simulink model "readArray2"  (R2012b)
settings: Solver=FixedStepDiscrete  SolverMode=MultiTasking  StartTime=0.0  StopTime=10.0  FixedStep=0.001  RelTol=1e-3
undefined symbols (not defined in the file): macaddr, modelConstants, mxpcnbunlink, rereferencingType
libraries: xpcnetworkbufferlib x2, xpcethernetlib x2, simulink x1
settings Model: xpc_rtwmakecfg_data=_xpcetherlib__xpcether8255xlib__xpcetherGbElib__xpcnblib_  BufferReuse=off  Creator=gilja  LastModifiedBy=NPTL
settings SolverCC: EnableConcurrentExecution=on  ConcurrentTasks=on
settings DataIOCC: SaveOutput=off  SignalLogging=off  DSMLogging=off  SaveTime=off
settings OptimizationCC: BlockReduction=off  InlineParams=on  InlineInvariantSignals=on  OptimizeBlockIOStorage=off  BufferReuse=off  ExpressionFolding=off  LocalBlockOutputs=off
settings HardwareCC: ProdIntDivRoundTo=Zero  ProdEndianess=LittleEndian  ProdHWDeviceType=Generic->32-bit x86 compatible
settings ModelReferenceCC: ModelReferenceNumInstancesAllowed=Single  PropagateVarSize=During execution  ModelReferenceMinAlgLoopOccurrences=on
settings SFSimCC: SimCustomHeaderCode="#include \"cerebusParse.h\""  SimUserSources=cerebusParse.c  SimUserIncludeDirs=C:\Progra~1\MATLAB\R2012b\toolbox\rtw\targets\xpc\target\build\xpcblocks\include
settings RTWCC: SystemTargetFile=xpctarget.tlc  TemplateMakefile=xpc_default_tmf  Description=xPC Target  ProcessScript=xpctarget_make_rtw_hook  RTWUseSimCustomCode=on  CustomHeaderCode="#include \"cerebusParse.h\""  CustomInclude=C:\Progra~1\MATLAB\R2012b\toolbox\rtw\targets\xpc\target\build\xpcblocks\include  CustomSource=cerebusParse.c  RTWCompilerOptimization=On
settings CodeAppCC: MaxIdLength=62
settings xpcTargetCC: TargetFcnLib=ansi_tfl_table_tmw.mat  CodeReplacementLibrary=XPC_BLAS  ParMdlRefBuildCompliant=on  ConcurrentExecutionCompliant=on  CombineSignalStateStructs=off  GRTInterface=on  xPCTaskExecutionProfile=on  xPCRL32EventNumber=5000  xPCisDownloadable=off  xPCLoadParamSetFile=off  xPCConcurrentTasks=off  xPCEnableSFAnimation=off

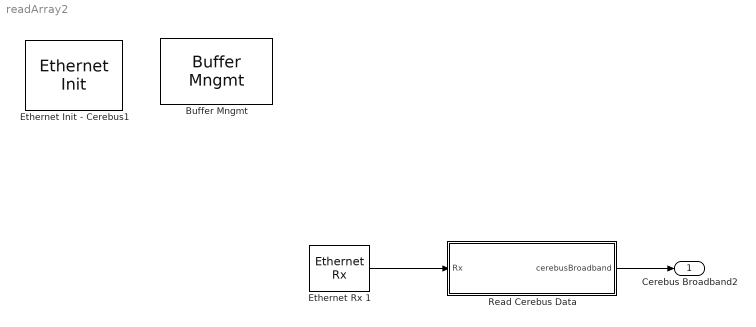
== system readArray2 ==
  "Buffer Mngmt " : xpcnetworkbufferlib/Buffer Mngmt   Priority=-1  SampleTime=-1  PoolSizes=modelConstants.networkBufferPoolSizes  ShowTune=on
  Ethernet Init - Cerebus1 : xpcethernetlib/Ethernet Init   Priority=-1  ID=5  Driver=Intel Gigabit  Bus=modelConstants.xpcNICConfig.nsp2.bus  Slot=modelConstants.xpcNICConfig.nsp2.slot  SampleTime=-1  AddressSource=Specify  MAC=macaddr('00:00:00:00:00:00')  TxSA=off  RxPromiscuous=off  Multicast={}  RxBad=off  RxShort=off  MaxMTU=1518  TxThreshold=10  TxBuffers=128  RxBuffers=64  ShowTune=on  NumRxBlks=1
  Ethernet Rx 1 : xpcethernetlib/Ethernet Rx   ID=5  SampleTime=modelConstants.sampleTime  Criteria=Receive all unmatched types [0 to 65535]  EtherType=[hex2dec('0000')]  BlkID=0
  Read Cerebus Data : Subsystem
  Cerebus Broadband2 : Outport  OutDataTypeStr=Bus: cerebusBroadband  BusOutputAsStruct=on
  wires:
  Ethernet Rx 1/1 -> Read Cerebus Data/1(Rx)
  Read Cerebus Data/1(cerebusBroadband) -> Cerebus Broadband2/1

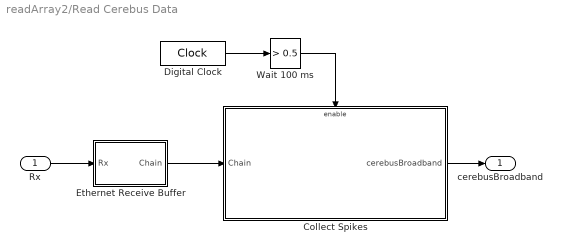
== system readArray2/Read Cerebus Data ==
  Rx : Inport
  Collect Spikes : Subsystem
  Digital Clock : DigitalClock  SampleTime=0.001
  Ethernet Receive Buffer : Subsystem
  Wait 100 ms : simulink/Logic and Bit Operations/Compare To Constant  relop=>  const=0.5  OutDataTypeStr=boolean
  cerebusBroadband : Outport  OutDataTypeStr=Bus: cerebusBroadband
  wires:
  Collect Spikes/1(cerebusBroadband) -> cerebusBroadband/1
  Wait 100 ms/1 -> Collect Spikes/Enable
  Digital Clock/1 -> Wait 100 ms/1
  Ethernet Receive Buffer/1(Chain) -> Collect Spikes/1(Chain)
  Rx/1 -> Ethernet Receive Buffer/1(Rx)

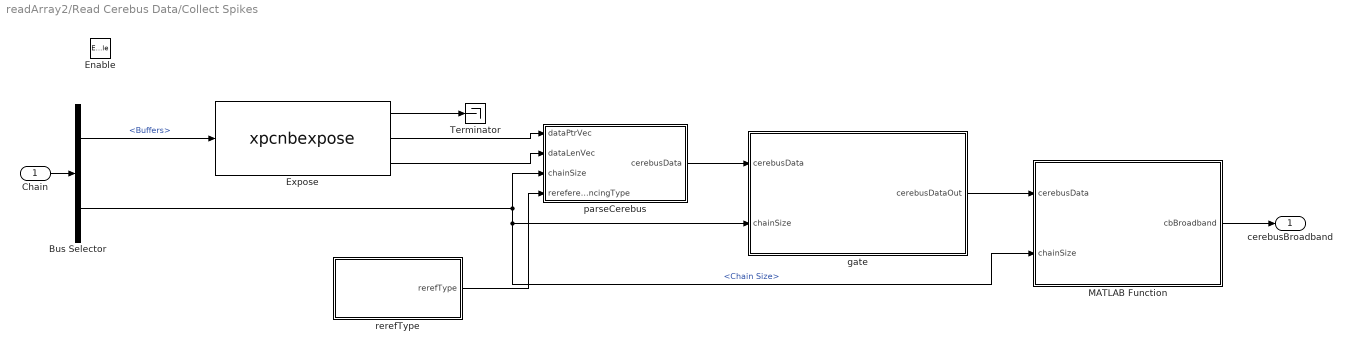
== system readArray2/Read Cerebus Data/Collect Spikes ==
  Chain : Inport
  Enable : EnablePort  StatesWhenEnabling=reset  PropagateVarSize=During execution
  Bus Selector : BusSelector  OutputSignals=Buffers,Chain Size
  Expose : S-Function  InitFcn=mxpcnbunlink(1,0);  FunctionName=xpcnbexpose  Parameters=vectorLength  EnableBusSupport=off  mask(xpcnbunlink){VectorLength=50}
      mask prompts: VectorLength "Vector length (-1 inherit):"
      mask help: Network Buffer Exposure
      mask init:
      | [vectorLength] = mxpcnbunlink(2, VectorLength);
      mask Help: eval('xpcdoc(''NB_Unlink'')');
      mask Display:
      | disp('NB Expose');
      | port_label('output', 1, 'NBVec');
      | port_label('output', 2, 'DataPtrVec');
      | port_label('output', 3, 'DataLenVec');
  MATLAB Function : MATLAB Function  TreatAsAtomicUnit=on
  Terminator : Terminator
  gate : MATLAB Function  TreatAsAtomicUnit=on
  parseCerebus : MATLAB Function  TreatAsAtomicUnit=on
  rerefType : Subsystem
  cerebusBroadband : Outport  OutDataTypeStr=Bus: cerebusBroadband
  wires:
  gate/1(cerebusDataOut) -> MATLAB Function/1(cerebusData)
  Chain/1 -> Bus Selector/1
  MATLAB Function/1(cbBroadband) -> cerebusBroadband/1
  Bus Selector/1 -> Expose/1  "<Buffers>"
  Expose/2 -> parseCerebus/1(dataPtrVec)
  Expose/3 -> parseCerebus/2(dataLenVec)
  Bus Selector/2 -> parseCerebus/3(chainSize), MATLAB Function/2(chainSize), gate/2(chainSize)  "<Chain Size>"
  parseCerebus/1(cerebusData) -> gate/1(cerebusData)
  Expose/1 -> Terminator/1
  rerefType/1(rerefType) -> parseCerebus/4(rereferencingType)

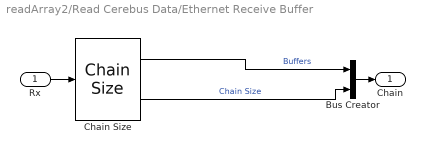
== system readArray2/Read Cerebus Data/Ethernet Receive Buffer ==
  Rx : Inport
  Bus Creator : BusCreator  Inputs=2
  "Chain Size " : xpcnetworkbufferlib/Chain Size 
  Chain : Outport
  wires:
  Rx/1 -> "Chain Size "/1
  "Chain Size "/2 -> Bus Creator/2  "Chain Size"
  Bus Creator/1 -> Chain/1
  "Chain Size "/1 -> Bus Creator/1  "Buffers"

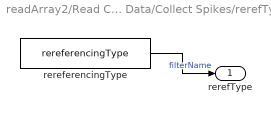
== system readArray2/Read Cerebus Data/Collect Spikes/rerefType ==
  rereferencingType : Constant  Value=rereferencingType
  rerefType : Outport
  wires:
  rereferencingType/1 -> rerefType/1  "filterName"

== matlab function readArray2/Read Cerebus Data/Collect Spikes/parseCerebus ==
  data: dataPtrVec input size=[1 50]; cerebusData output Bus: cerebusData; dataLenVec input size=[1 50]; chainSize input size=[1 1]; rereferencingType input
function cerebusData  = parseCerebus(dataPtrVec, dataLenVec, chainSize, rereferencingType)
%#codegen

    persistent lastPacketTime;
    persistent firstPacket;
    persistent contiguousInvalidGroupPackets;
    if isempty(lastPacketTime)
        lastPacketTime = uint32(0);
        firstPacket = true;
        contiguousInvalidGroupPackets = uint16(0);
    end

    %numCerebusChannels = xpcConstants.cerebus.numCerebusChannels;
    %maxSamplesInMS = xpcConstants.cerebus.maxSamplesInMS;
    %continuousGroupId = xpcConstants.cerebus.continuousGroupId;
    
    numCerebusChannels = 96;
    maxSamplesInMS = 150;
    continuousGroupId = 5;
    
    % initialize
    numSamples = uint32(0); % ideally, either 0, 30, or 60
    samples = zeros([numCerebusChannels maxSamplesInMS], 'int16');
    cerebusTimes = zeros(maxSamplesInMS, 1, 'uint32');
    
    curTime = coder.nullcopy(uint32(0));
    
    %% 
    % loop through all UDP packets that came in
    for iP = uint8(1) : uint8(chainSize)
        
        if dataPtrVec(iP) == 0 || dataLenVec(iP) == 0
            continue;
        end

        % define buffers
        pp = coder.opaque('cbPKT_GENERIC*', 'NULL');
        pBufferEnd = coder.opaque('UINT8_T*', 'NULL');
        
        % grab pointer to end of UDP packet
        pp = coder.ceval('(cbPKT_GENERIC*)', dataPtrVec(iP) + uint32(42)); % do a cast operation - +42 is for jumping over the ethernet + IP + UDP header
        pBufferEnd = coder.ceval('cb_getPointerToBufferEnd', pp, uint32(dataLenVec(iP)));
        
        %%
        % loop over all cbPkts in this UDP packet
        while true  


            isGroupPkt = coder.nullcopy(uint8(0));
            isGroupPkt = coder.ceval('cb_isContinuousPacketForGroup', pp, uint8(continuousGroupId));
                       
            if isGroupPkt
                
                % get time
                curTime = coder.nullcopy(uint32(0));
                curTime = coder.ceval('cb_getTime', pp); % uint32 cerebus timestamp

                % CP & PN - 16/09/20 avoiding bad group packets that seem to pass
                % groupId screen, yet have very odd sample times
                if firstPacket
                    firstPacket = false;
                    lastPacketTime = curTime; % last valid uint32 timestamp
                else
                    % if the packet has a weird timestamp, do not increment
                    % numsamples, do not copy into continuous samples
                    if abs( single(curTime) - single(lastPacketTime) ) < 61 % we can drop 2 ms of packets, and this screen still works
                        
                        % receieved continuous data sample for the appropriate group id
                        numSamples = numSamples + uint32(1);
                        contiguousInvalidGroupPackets = uint16(0);
                        lastPacketTime = curTime;

                        cerebusTimes(numSamples) = curTime;

                        % copy in the samples
                        coder.ceval('cb_copyContinuousSamples', pp, coder.ref(samples(1, numSamples)), size(samples, 1)); 
                        
                    else
                        
                        % got invalid group packet
                        contiguousInvalidGroupPackets = contiguousInvalidGroupPackets + uint16(1);
                        
                    end
                end
                
            end
            
            % test to ensure we didn't get a bad timestamp on the very
            % first time, otherwise will never get neural data
            if contiguousInvalidGroupPackets > uint16(100)
                contiguousInvalidGroupPackets = uint16(0);
                lastPacketTime = curTime;
            end

            % jump to the next cbPKT
            pNext = coder.nullcopy(uint8(0));
            pNext = coder.ceval('cb_hasNext', pp, pBufferEnd);
            
            if ~pNext % check to see if no more cbPkts in this UDP packet
                break; % break while
            end
            
            % update pointer to next cbPkt
            pNext = coder.opaque('cbPKT_GENERIC*', 'NULL');
            pNext = coder.ceval('cb_getNext', pp);
            pp = pNext;
            
        end  % end while loop over all cbPkts in this UDP packet
        
    end % end for loop over all UDP packets

    % apply rereferencing
    switch rereferencingType
        case rigHardwareConstants.REREFERENCE_NONE
            % no common referencing, take the values as is, do nothing here
        case rigHardwareConstants.REREFERENCE_COMMON_AVG
            % Common avg reference:
            samples(:,1:numSamples) = samples(:,1:numSamples) - int16( repmat(   mean(single(samples(:, 1:numSamples)), 1), size(samples, 1), 1) );
        case rigHardwareConstants.REREFERENCE_COMMON_MEDIAN
            % Common median reference:
            samples(:,1:numSamples) = samples(:,1:numSamples) - int16( repmat( median(single(samples(:, 1:numSamples)), 1), size(samples, 1), 1) );
    end
    
    cerebusData.numSamples = numSamples;
    cerebusData.samples = samples'; % this is time x channels
    cerebusData.sampleTimes = cerebusTimes;
    cerebusData.firstCerebusTime = cerebusTimes(1);
    cerebusData.lastCerebusTime = cerebusTimes(numSamples);

end

== matlab function readArray2/Read Cerebus Data/Collect Spikes/MATLAB Function ==
  data: cerebusData input Bus: cerebusData; cbBroadband output Bus: cerebusBroadband size=1; xpcConstants parameter; chainSize input size=[1 1]
function cbBroadband  = bufferCerebusSamples(cerebusData, xpcConstants, chainSize)
%#codegen

persistent sampleBuffer bufferInIdx bufferOutIdx outputValidP bufferInit;

numCerebusChannels = xpcConstants.cerebus.numCerebusChannels;
bufferSize = xpcConstants.cerebus.sampleBufferSize;
bufferDelay = xpcConstants.cerebus.sampleBufferDelay;


if(isempty(sampleBuffer))
    sampleBuffer = int16(zeros(bufferSize, numCerebusChannels));
    bufferInIdx = 0;
    bufferOutIdx = bufferSize;
    outputValidP = false;
    bufferInit = true;
end

cerebusFrame = int16(zeros(30, numCerebusChannels));

if(bufferInIdx < bufferOutIdx)
    bufferSpace = bufferOutIdx - bufferInIdx;
else
    bufferSpace = bufferSize - bufferInIdx + bufferOutIdx;
end

if(cerebusData.numSamples > bufferSpace)
    bufferInit = false;
    outputValidP = false;
end

% if((cerebusData.numSamples > 0) && (cerebusData.numSamples < bufferSize))
%     sampleBuffer(bufferInIdx + [1:cerebusData.numSamples], :) = cerebusData.samples(1:cerebusData.numSamples, :);
%     bufferInIdx = mod((bufferInIdx + double(cerebusData.numSamples)), bufferSize);
% end

if((cerebusData.numSamples > 0) && (cerebusData.numSamples < bufferSpace))
    for nn = 1:cerebusData.numSamples
        indx= 1+mod(double(bufferInIdx + nn)-1, bufferSize);
        sampleBuffer(indx, :) = cerebusData.samples(nn, :);
    end
    bufferInIdx = mod((bufferInIdx + double(cerebusData.numSamples)), bufferSize);
end

if(bufferInit)
    if(bufferInIdx >= (bufferDelay))
        bufferInit = false;
        outputValidP = true;
    end
elseif(outputValidP)
    numToEndOfBuffer = bufferSize - bufferOutIdx;
    if( (numToEndOfBuffer >= 30) && ...
            ((bufferInIdx >= bufferOutIdx + 30) || (bufferInIdx < bufferOutIdx)) )
        cerebusFrame = sampleBuffer(bufferOutIdx+[1:30], :);
        
    elseif ( (numToEndOfBuffer < 30) ...
            && (bufferInIdx >= (30 - numToEndOfBuffer) ))
        idx = [1:30];
        idx(1:numToEndOfBuffer) = idx(1:numToEndOfBuffer) + bufferOutIdx;
        idx(numToEndOfBuffer+1:end) = idx(numToEndOfBuffer+1:end) - numToEndOfBuffer;
        cerebusFrame = sampleBuffer(idx, :);
        
    else
        outputValidP = false;
    end
    
    bufferOutIdx = mod((bufferOutIdx + 30), bufferSize);
end

cbBroadband.cerebusFrame = cerebusFrame;
cbBroadband.outputValid = outputValidP;
cbBroadband.firstCerebusTime = cerebusData.firstCerebusTime;
cbBroadband.lastCerebusTime = cerebusData.lastCerebusTime;
cbBroadband.sampleTimes = cerebusData.sampleTimes(1:50);
cbBroadband.numSamples = cerebusData.numSamples;
cbBroadband.chainSize = uint16(chainSize); %% this will be set downstream

end

== matlab function readArray2/Read Cerebus Data/Collect Spikes/gate ==
  data: cerebusData input Bus: cerebusData; chainSize input size=[1 1]; cerebusDataOut output Bus: cerebusData; xpcConstants parameter
function cerebusDataOut = checkNoPackets(cerebusData, chainSize, xpcConstants)


if chainSize == 0
    cerebusData.samples = coder.nullcopy(int16(zeros(xpcConstants.cerebus.maxSamplesInMS, xpcConstants.cerebus.numCerebusChannels)));
    cerebusData.sampleTimes = coder.nullcopy(uint32(zeros(xpcConstants.cerebus.maxSamplesInMS,1)));
    cerebusData.numSamples = uint32(0);
    
    cerebusData.firstCerebusTime = uint32(0);
    cerebusData.lastCerebusTime = uint32(0);
end

cerebusDataOut = cerebusData;
